simulink model "Model_to_SIL_Arduino"  (R2022b)
settings: Solver=ode3  StartTime=0.0  StopTime=10.0  FixedStep=0.01  RelTol=1e-3  EnableMultiTasking=on
values from neighbouring files (symbols this model uses):
  Acceleration_Max = 3.2    [Matlab_WorkSpace.mat]
  Distance_initial = 8    [Matlab_WorkSpace.mat]
  Frein_Max = -9    [Matlab_WorkSpace.mat]
  glissement = 0.22    [Matlab_WorkSpace.mat]
  r = 0.3    [Matlab_WorkSpace.mat]
  vehicule_half_length = 2.5    [Matlab_WorkSpace.mat]
libraries: arduinosensorlib x1, slpidlib x1
settings Model: ExtModeTrigDuration=2  Creator=Yoamiri  LastModifiedBy=Yoamiri
settings SolverCC: AutoInsertRateTranBlk=on
settings OptimizationCC: EnhancedBackFolding=on  PassReuseOutputArgsAs=Individual arguments  ZeroExternalMemoryAtStartup=off  ZeroInternalMemoryAtStartup=off  MaxStackSize=64  OptimizeBlockOrder=speed  DifferentSizesBufferReuse=on  OptimizationCustomize=off  EfficientTunableParamExpr=on
settings DebuggingCC: ParameterPrecisionLossMsg=none  ParameterTunabilityLossMsg=error
settings HardwareCC: ProdBitPerInt=16  ProdBitPerPointer=16  ProdBitPerSizeT=16  ProdBitPerPtrDiffT=16  ProdLargestAtomicFloat=None  ProdWordSize=8  ProdHWDeviceType=Atmel->AVR
settings SFSimCC: MATLABDynamicMemAlloc=off
settings RTWCC: Description=Embedded Coder  SystemTargetFile=ert.tlc  HardwareBoard=Arduino Uno  TLCOptions=-aInlineSetEventsForThisBaseRateFcn=TLC_FALSE -aSuppressMultiTaskScheduler=TLC_FALSE -aRateBasedStepFcn=1  TemplateMakefile=ert_default_tmf  Toolchain=Arduino AVR  BuildConfiguration=Faster Runs  PortableWordSizes=on  CreateSILPILBlock=PIL
settings CodeAppCC: ForceParamTrailComments=on  IgnoreCustomStorageClasses=off  OperatorAnnotations=on  SimulinkDataObjDesc=on  SFDataObjDesc=on  InsertBlockDesc=on
settings ERTTargetCC: SupportContinuousTime=on  SupportVariableSizeSignals=on  ExtModeTransport=3  ExtModeStaticAlloc=on  ExtModeAutomaticAllocSize=off  ExtModeStaticAllocSize=250  ExtModeMexFile=ext_xcp  ExtModeIntrfLevel=Level2 - Open

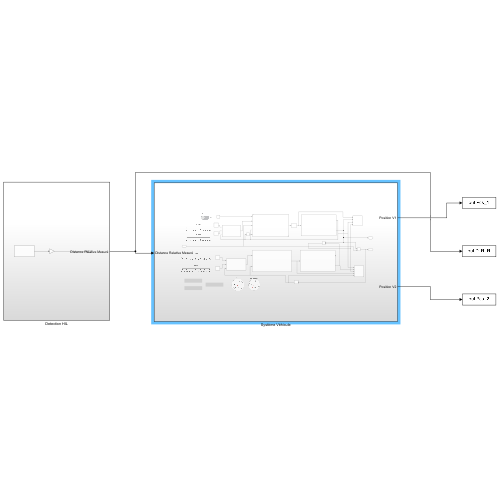
[thumbnail: Simulink's stored preview of the top-level diagram]
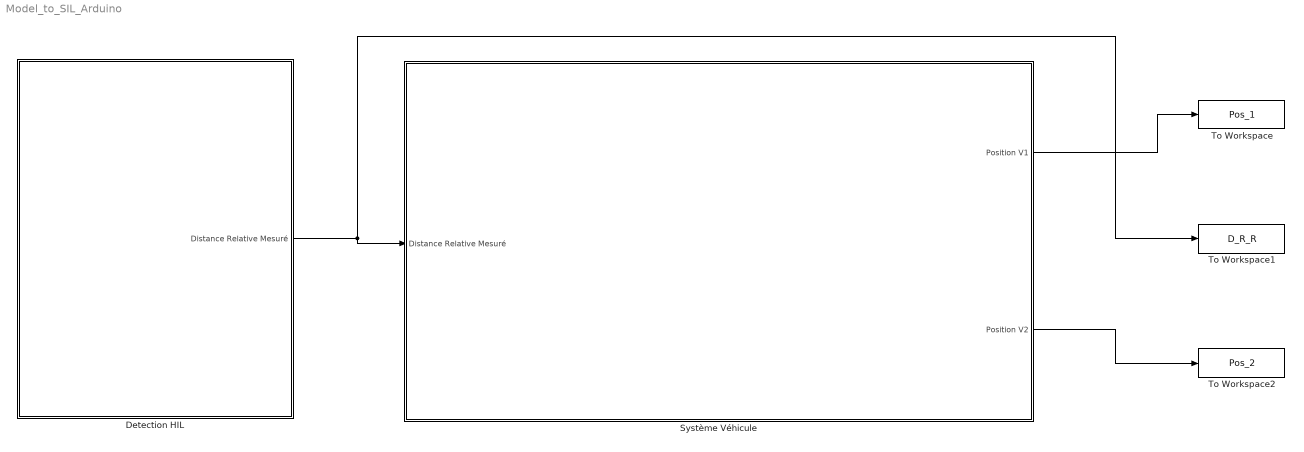
== system Model_to_SIL_Arduino ==
  Detection HIL : Subsystem
  Système Véhicule : Subsystem
  To Workspace : ToWorkspace  VariableName=Pos_1  SaveFormat=Structure With Time  SampleTime=0.01
  To Workspace1 : ToWorkspace  VariableName=D_R_R  SaveFormat=Structure With Time  SampleTime=0.01
  To Workspace2 : ToWorkspace  VariableName=Pos_2  SaveFormat=Structure With Time  SampleTime=0.01
  wires:
  Système Véhicule/2(Position V2) -> To Workspace2/1
  Système Véhicule/1(Position V1) -> To Workspace/1
  Detection HIL/1(Distance Relative Mesuré) -> To Workspace1/1, Système Véhicule/1(Distance Relative Mesuré)

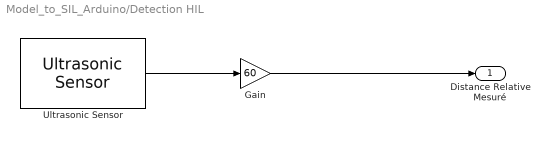
== system Model_to_SIL_Arduino/Detection HIL ==
  Gain : Gain  Gain=60
  Ultrasonic Sensor : arduinosensorlib/Ultrasonic Sensor  NumSignalPins=1  TrigPin=4  EchoPin=5  SignalPin=3  SampleTime_=0.1  blockPlatform=ARDUINO
  Distance Relative Mesuré : Outport
  wires:
  Ultrasonic Sensor/1 -> Gain/1
  Gain/1 -> Distance Relative Mesuré/1

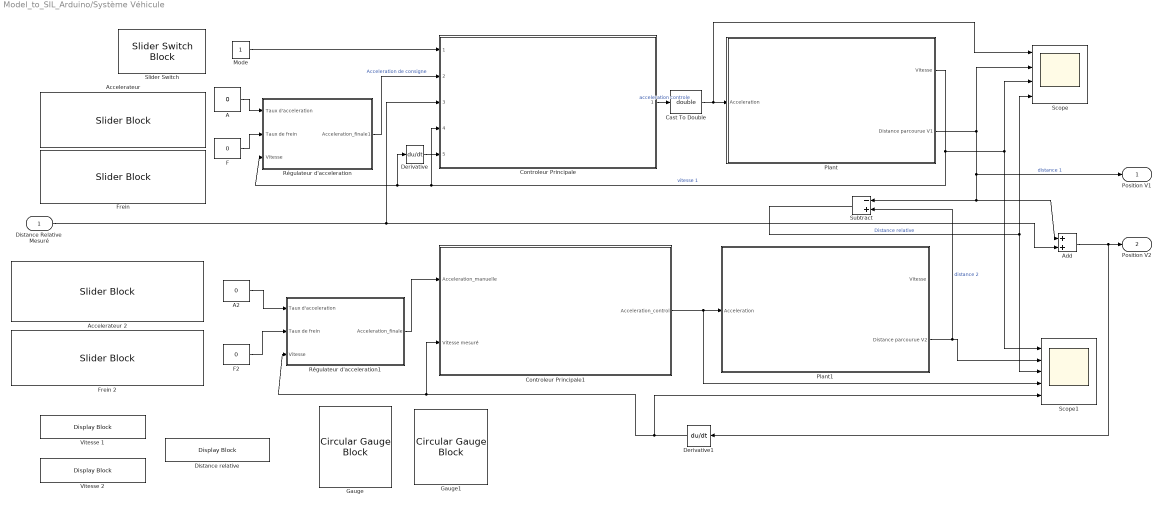
== system Model_to_SIL_Arduino/Système Véhicule ==
  Distance Relative Mesuré : Inport
  A : Constant  Value=0
  A2 : Constant  Value=0
  Accelerateur : SliderBlock
  Accelerateur 2 : SliderBlock  TickInterval=10
  Add : Sum
  Cast To Double : DataTypeConversion  OutDataTypeStr=double  SaturateOnIntegerOverflow=off  RndMeth=Floor
  Controleur Principale : Subsystem  TreatAsAtomicUnit=on  ReferencedSubsystem=Controleur_Principale_SIL
  Controleur Principale1 : Subsystem
  Derivative : Derivative
  Derivative1 : Derivative
  Distance relative : DisplayBlock  LabelPosition=Hide  Transparency=1
  F : Constant  Value=0
  F2 : Constant  Value=0
  Frein : SliderBlock
  Frein 2 : SliderBlock  TickInterval=10
  Gauge : CircularGaugeBlock
  Gauge1 : CircularGaugeBlock
  Mode : Constant  OutDataTypeStr=boolean
  Plant : Subsystem
  Plant1 : Subsystem
  Régulateur d'acceleration : Subsystem
  Régulateur d'acceleration1 : Subsystem
  Scope : Scope  NumInputPorts=4
  Scope1 : Scope  NumInputPorts=5
  Slider Switch : SliderSwitchBlock
      settings: Values={{'Off', 'On'}, [1 0]}
  Subtract : Sum  Inputs=-+
  Vitesse 1 : DisplayBlock  LabelPosition=Hide  Transparency=1
  Vitesse 2 : DisplayBlock  LabelPosition=Hide  Transparency=1
  Position V1 : Outport
  Position V2 : Outport  Port=2
  wires:
  Controleur Principale1/1(Acceleration_control) -> Plant1/1(Acceleration), Scope1/4
  A2/1 -> Régulateur d'acceleration1/1(Taux d'acceleration)
  Régulateur d'acceleration1/1(Acceleration_finale) -> Controleur Principale1/1(Acceleration_manuelle)
  Régulateur d'acceleration/1(Acceleration_finale1) -> Controleur Principale/2  "Acceleration de consigne"
  Controleur Principale/1 -> Cast To Double/1  "acceleration controle"
  F2/1 -> Régulateur d'acceleration1/2(Taux de frein)
  Plant/1(Vitesse) -> Scope/3, Scope1/1, Controleur Principale/4, Derivative/1, Régulateur d'acceleration/3(Vitesse)  "vitesse 1"
  Mode/1 -> Controleur Principale/1
  Subtract/1 -> Scope/4, Scope1/3  "Distance relative"
  Plant/2(Distance parcourue V1) -> Add/1, Subtract/1, Position V1/1, Scope/2  "distance 1"
  Plant1/2(Distance parcourue V2) -> Scope1/2, Subtract/2  "distance 2"
  A/1 -> Régulateur d'acceleration/1(Taux d'acceleration)
  F/1 -> Régulateur d'acceleration/2(Taux de frein)
  Distance Relative Mesuré/1 -> Controleur Principale/3, Add/2
  Cast To Double/1 -> Scope/1, Plant/1(Acceleration)
  Derivative/1 -> Controleur Principale/5
  Add/1 -> Derivative1/1, Position V2/1
  Derivative1/1 -> Scope1/5, Controleur Principale1/2(Vitesse mesuré), Régulateur d'acceleration1/3(Vitesse)

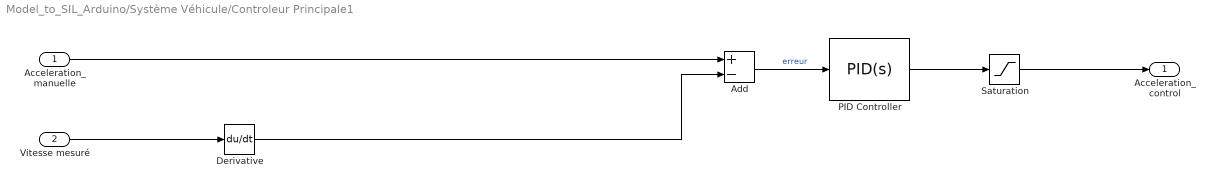
== system Model_to_SIL_Arduino/Système Véhicule/Controleur Principale1 ==
  Acceleration_manuelle : Inport
  Vitesse mesuré : Inport  Port=2
  Add : Sum  Inputs=+-
  Derivative : Derivative
  PID Controller : slpidlib/PID Controller  Controller=PID  Form=Parallel  TimeDomain=Continuous-time  UseExternalTs=off  SampleTime=-1  IntegratorMethod=Forward Euler  FilterMethod=Forward Euler  ControllerParametersSource=internal  P=4  I=1.5  UseKiTs=off  D=0  N=100  UseFilter=on  TunerSelectOption=Transfer Function Based (PID Tuner App)  InitialConditionSource=internal  InitialConditionForIntegrator=0  InitialConditionForFilter=0  DifferentiatorICPrevScaledInput=0  ExternalReset=none  TrackingMode=off  Kt=1  LimitOutput=off  SatLimitsSource=internal  UpperSaturationLimit=inf  LowerSaturationLimit=-inf  LinearizeAsGain=on  AntiWindupMode=none  Kb=1  LimitIntegrator=off  UpperIntegratorSaturationLimit=inf  LowerIntegratorSaturationLimit=-inf  POutMin=[]  POutMax=[]  IOutMin=[]  IOutMax=[]  DOutMin=[]  DOutMax=[]  NOutMin=[]  NOutMax=[]  SumOutMin=[]  SumOutMax=[]  SaturationOutMin=[]  SaturationOutMax=[]  PParamMin=[]  PParamMax=[]  IParamMin=[]  IParamMax=[]  DParamMin=[]  DParamMax=[]  NParamMin=[]  NParamMax=[]  KbParamMin=[]  KbParamMax=[]  KtParamMin=[]  KtParamMax=[]  KbOutMin=[]  KbOutMax=[]  KtOutMin=[]  KtOutMax=[]  IntegratorOutMin=[]  IntegratorOutMax=[]  FilterOutMin=[]  FilterOutMax=[]  SumI1OutMin=[]  SumI1OutMax=[]  SumI2OutMin=[]  SumI2OutMax=[]  SumI3OutMin=[]  SumI3OutMax=[]  SumI4OutMin=[]  SumI4OutMax=[]  SumDOutMin=[]  SumDOutMax=[]  DifferentiatorOutMin=[]  DifferentiatorOutMax=[]  FilterDiffOutCoefMin=[]  FilterDiffOutCoefMax=[]  ReciprocalOutMin=[]  ReciprocalOutMax=[]  SumDenOutMin=[]  SumDenOutMax=[]  SumNumOutMin=[]  SumNumOutMax=[]  DivideOutMin=[]  DivideOutMax=[]  UdiffTsProdOutMin=[]  UdiffTsProdOutMax=[]  NTsProdOutMin=[]  NTsProdOutMax=[]  UintegralTsProdOutMin=[]  UintegralTsProdOutMax=[]  UngainTsProdOutMin=[]  UngainTsProdOutMax=[]  ClampingZeroOutDataTypeStr=Inherit: Inherit via back propagation  ClampingZeroOutMin=[]  ClampingZeroOutMax=[]  FilterDenConstantOutDataTypeStr=Inherit: Inherit via back propagation  FilterDenConstantOutMin=[]  FilterDenConstantOutMax=[]  PCopyOutDataTypeStr=Inherit: Inherit via back propagation  PCopyOutMin=[]  PCopyOutMax=[]  NCopyOutDataTypeStr=Inherit: Inherit via back propagation  NCopyOutMin=[]  NCopyOutMax=[]  IntegratorContinuousStateAttributes=''  IntegratorStateMustResolveToSignalObject=off  IntegratorRTWStateStorageClass=Auto  FilterContinuousStateAttributes=''  FilterStateMustResolveToSignalObject=off  FilterRTWStateStorageClass=Auto  ParallelPVariant=InternalParameters  IdealPVariant=Disabled  IVariant=InternalParameters  DVariant=InternalParameters  IntegratorVariant=Continuous  SatVariant=Disabled  AWVariant=Passthrough  PCopyVariant=Disabled  TRVariant=Disabled  FdbkBlocksVariant=Forward  IdealPFdbkVariant=Disabled  SatFdbkVariant=Disabled  DerivativeFilterVariant=ContFilter  NVariant=InternalParameters  NCopyVariant=Disabled  FilterICVariant=InternalICsFilter  IntegratorICVariant=InternalICs  ExternalResetVariant=Disabled  TRSumVariant=Passthrough  SumFdbkVariant=Disabled  SumVariant=Sum_PID  TsampFilterVariant=InternalTs  TsampNgainVariant=Passthrough  TsampIntegralVariant=Passthrough  ExternalSaturationOutDataTypeStr=Inherit: Same as second input
  Saturation : Saturate  UpperLimit=Acceleration_Max  LowerLimit=Frein_Max
  Acceleration_control : Outport
  wires:
  Vitesse mesuré/1 -> Derivative/1
  Derivative/1 -> Add/2
  Add/1 -> PID Controller/1  "erreur"
  PID Controller/1 -> Saturation/1
  Acceleration_manuelle/1 -> Add/1
  Saturation/1 -> Acceleration_control/1

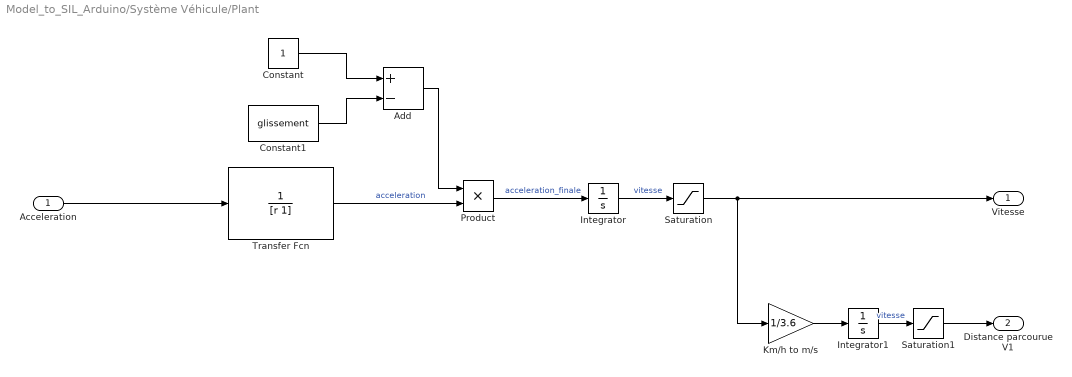
== system Model_to_SIL_Arduino/Système Véhicule/Plant ==
  Acceleration : Inport
  Add : Sum  Inputs=+-
  Constant : Constant
  Constant1 : Constant  Value=glissement
  Integrator : Integrator
  Integrator1 : Integrator
  Km/h to m/s : Gain  Gain=1/3.6
  Product : Product
  Saturation : Saturate  UpperLimit=120  LowerLimit=0
  Saturation1 : Saturate  UpperLimit=inf  LowerLimit=0
  Transfer Fcn : TransferFcn  Denominator=[r 1]
  Vitesse : Outport
  Distance parcourue V1 : Outport  Port=2
  wires:
  Acceleration/1 -> Transfer Fcn/1
  Product/1 -> Integrator/1  "acceleration_finale"
  Transfer Fcn/1 -> Product/2  "acceleration"
  Constant/1 -> Add/1
  Constant1/1 -> Add/2
  Add/1 -> Product/1
  Integrator1/1 -> Saturation1/1  "vitesse"
  Saturation/1 -> Vitesse/1, Km/h to m/s/1
  Saturation1/1 -> Distance parcourue V1/1
  Km/h to m/s/1 -> Integrator1/1
  Integrator/1 -> Saturation/1  "vitesse"

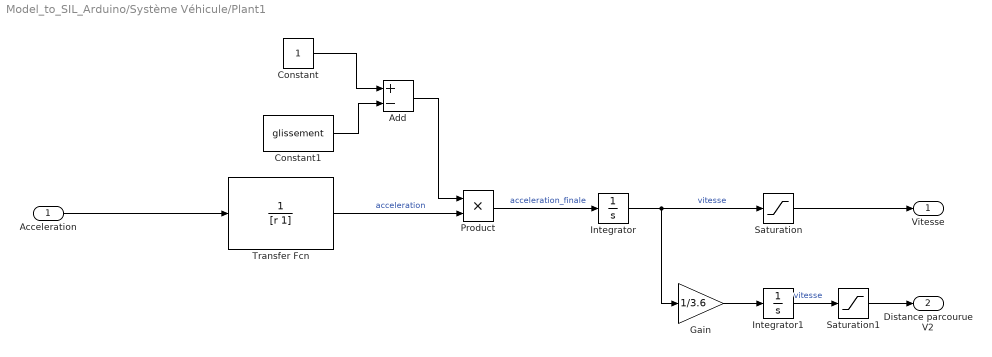
== system Model_to_SIL_Arduino/Système Véhicule/Plant1 ==
  Acceleration : Inport
  Add : Sum  Inputs=+-
  Constant : Constant
  Constant1 : Constant  Value=glissement
  Gain : Gain  Gain=1/3.6
  Integrator : Integrator
  Integrator1 : Integrator  InitialCondition=Distance_initial+vehicule_half_length
  Product : Product
  Saturation : Saturate  UpperLimit=120  LowerLimit=0
  Saturation1 : Saturate  UpperLimit=inf  LowerLimit=0
  Transfer Fcn : TransferFcn  Denominator=[r 1]
  Vitesse : Outport
  Distance parcourue V2 : Outport  Port=2
  wires:
  Acceleration/1 -> Transfer Fcn/1
  Product/1 -> Integrator/1  "acceleration_finale"
  Transfer Fcn/1 -> Product/2  "acceleration"
  Constant/1 -> Add/1
  Constant1/1 -> Add/2
  Add/1 -> Product/1
  Integrator/1 -> Saturation/1, Gain/1  "vitesse"
  Integrator1/1 -> Saturation1/1  "vitesse"
  Gain/1 -> Integrator1/1
  Saturation/1 -> Vitesse/1
  Saturation1/1 -> Distance parcourue V2/1

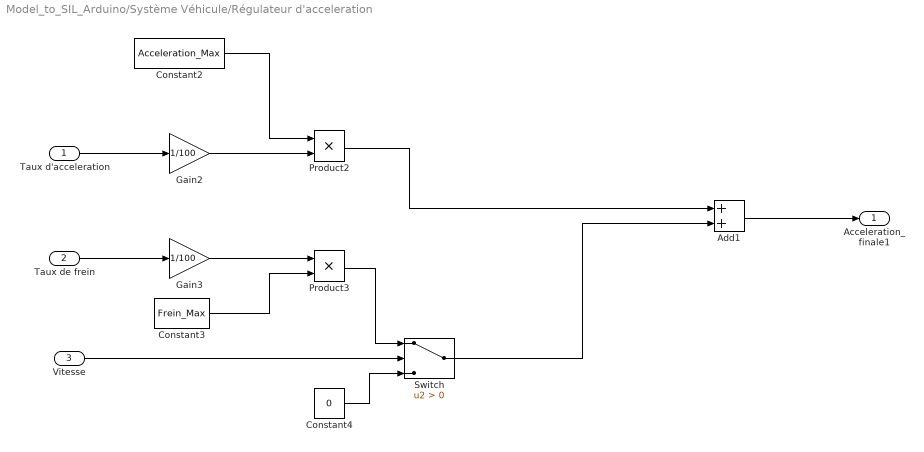
== system Model_to_SIL_Arduino/Système Véhicule/Régulateur d'acceleration ==
  Taux d'acceleration : Inport
  Taux de frein : Inport  Port=2
  Vitesse : Inport  Port=3
  Add1 : Sum
  Constant2 : Constant  Value=Acceleration_Max
  Constant3 : Constant  Value=Frein_Max
  Constant4 : Constant  Value=0
  Gain2 : Gain  Gain=1/100
  Gain3 : Gain  Gain=1/100
  Product2 : Product
  Product3 : Product
  Switch : Switch  Criteria=u2 > Threshold  SaturateOnIntegerOverflow=off  InputSameDT=off
  Acceleration_finale1 : Outport
  wires:
  Constant4/1 -> Switch/3
  Product3/1 -> Switch/1
  Vitesse/1 -> Switch/2
  Switch/1 -> Add1/2
  Product2/1 -> Add1/1
  Taux d'acceleration/1 -> Gain2/1
  Gain3/1 -> Product3/1
  Add1/1 -> Acceleration_finale1/1
  Constant2/1 -> Product2/1
  Taux de frein/1 -> Gain3/1
  Gain2/1 -> Product2/2
  Constant3/1 -> Product3/2

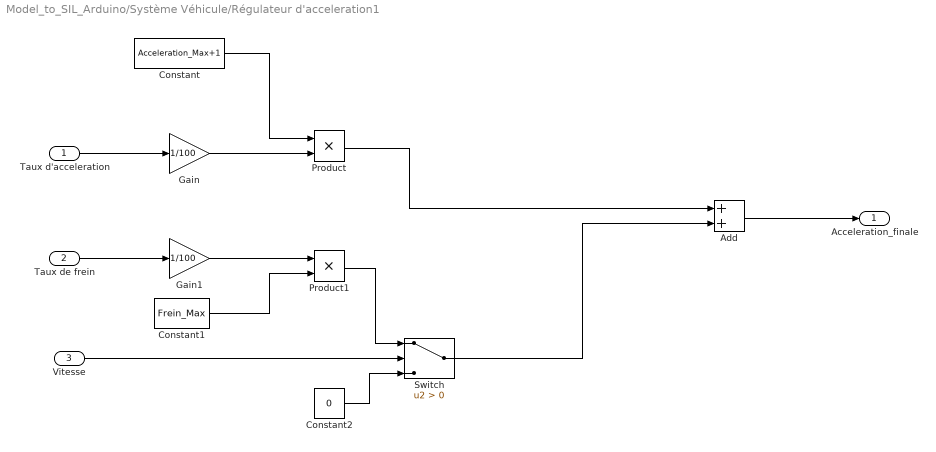
== system Model_to_SIL_Arduino/Système Véhicule/Régulateur d'acceleration1 ==
  Taux d'acceleration : Inport
  Taux de frein : Inport  Port=2
  Vitesse : Inport  Port=3
  Add : Sum
  Constant : Constant  Value=Acceleration_Max+1
  Constant1 : Constant  Value=Frein_Max
  Constant2 : Constant  Value=0
  Gain : Gain  Gain=1/100
  Gain1 : Gain  Gain=1/100
  Product : Product
  Product1 : Product
  Switch : Switch  Criteria=u2 > Threshold  SaturateOnIntegerOverflow=off  InputSameDT=off
  Acceleration_finale : Outport
  wires:
  Taux de frein/1 -> Gain1/1
  Taux d'acceleration/1 -> Gain/1
  Constant1/1 -> Product1/2
  Constant/1 -> Product/1
  Gain/1 -> Product/2
  Gain1/1 -> Product1/1
  Product/1 -> Add/1
  Add/1 -> Acceleration_finale/1
  Vitesse/1 -> Switch/2
  Product1/1 -> Switch/1
  Switch/1 -> Add/2
  Constant2/1 -> Switch/3
